simulink model "sds1104receiver"  (R2023a)
settings: Solver=VariableStepAuto  StartTime=0.0  StopTime=inf  RelTol=1e-3
settings Model: Creator=User  LastModifiedBy=User

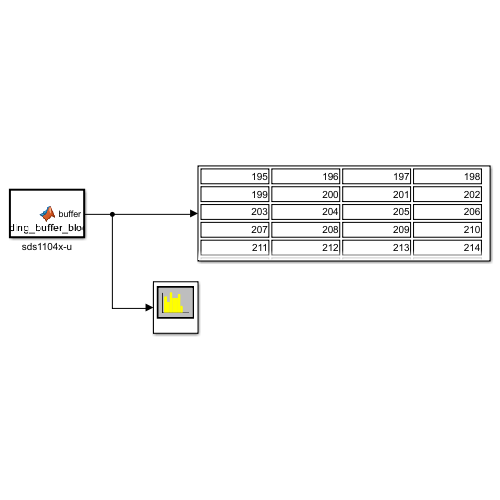
[thumbnail: Simulink's stored preview of the top-level diagram]
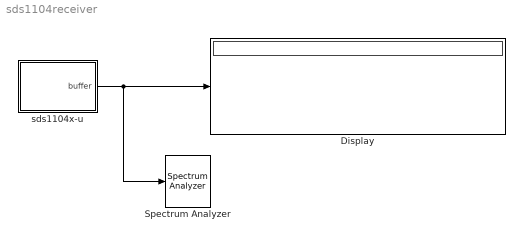
== system sds1104receiver ==
  Display : Display
  Spectrum Analyzer : SpectrumAnalyzer  WindowPosition=[2063.000000,389.000000,800.000000,500.000000,]  Visible=on  ScopeFrameLocation=window  SampleRateSource=Property  SampleRate=44.1e3  PlotAsTwoSidedSpectrum=off  FrequencyScale=Log  FrequencySpan=Start and stop frequencies  StartFrequency=20  StopFrequency=20e3  YLimits=[-187.41995798,100.94688694]  ColorLimits=[-20 80]  DefaultConfigurationName=spbscopes.SpectrumAnalyzerBlockCfg  IsFrequencyInputMode=0  FrequencyVectorPort=0  FrequencyVectorFromPort=0  FrequencyInputRBWPort=0  FrequencyInputRBWFromPort=0
  sds1104x-u : MATLAB Function  TreatAsAtomicUnit=on
  wires:
  sds1104x-u/1(buffer) -> Spectrum Analyzer/1, Display/1

== matlab function sds1104receiver/sds1104x-u ==
  data: buffer output
% this is for simulink matlab module
function buffer = read_file_from_oscilloscope_receiver()
    persistent buf
    if isempty(buf)
        buf = zeros(1024,1,'uint8');
    end
    buffer = zeros(1024,1,'uint8');
    % Call helper function to get latest data
    buf = read_file_helper();
    buffer(:) = buf(:);
end
